simulink model "W_integ_oClientServer_Model"  (R2024b)
settings: Solver=FixedStepDiscrete  StartTime=0.0  StopTime=10.0  FixedStep=0.05  RelTol=1e-3
undefined symbols (not defined in the file or in its folder): call_ServerService_getDataC, call_ServerService_setDataA, call_ServerService_setDataB
settings Model: Tag=EP_AA_WRAPPER_INTEGRATION  DataDictionary=Wrapper_oClientServer_Model.sldd  Creator=nabilekhoury  LastModifiedBy=nabilekhoury
settings OptimizationCC: DefaultParameterBehavior=Inlined  OptimizeBlockIOStorage=off  BufferReuse=off  ReuseModelBlockBuffer=off  GlobalBufferReuse=off  ExpressionFolding=off  EnableMemcpy=off  PassReuseOutputArgsAs=Individual arguments  LocalBlockOutputs=off  ZeroExternalMemoryAtStartup=off  ZeroInternalMemoryAtStartup=off  OptimizeDataStoreBuffers=off  BusAssignmentInplaceUpdate=off  OptimizationLevel=level0  OptimizationCustomize=off  EfficientTunableParamExpr=on
settings DebuggingCC: ParameterTunabilityLossMsg=error
settings ModelReferenceCC: ModelReferenceNumInstancesAllowed=Single
settings SFSimCC: MATLABDynamicMemAlloc=off  SimTargetLang=C++
settings RTWCC: Description=Embedded Coder  SystemTargetFile=ert.tlc  GenCodeOnly=on  TemplateMakefile=ert_default_tmf  CustomSourceCode="#include \"oClientServer_Model_adapter.h\""  CustomInitializer=sut_initialize();  TargetLang=C++
settings CodeAppCC: ForceParamTrailComments=on  IgnoreCustomStorageClasses=off  MaxIdLength=256  OperatorAnnotations=on  SimulinkDataObjDesc=on  SFDataObjDesc=on  CustomSymbolStrGlobalVar=w_$R$N$M  CustomSymbolStrType=w_$N$R$M_T  InsertBlockDesc=on
settings ERTTargetCC: TargetLangStandard=C++17 (ISO)  GenerateSampleERTMain=on  SupportAbsoluteTime=off  SupportNonFinite=off  SupportComplex=off  RootIOFormat=Structure reference  ERTCustomFileTemplate=example_file_process.tlc

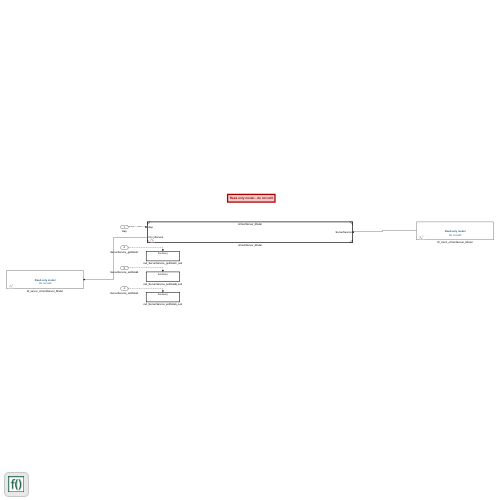
[thumbnail: Simulink's stored preview of the top-level diagram]
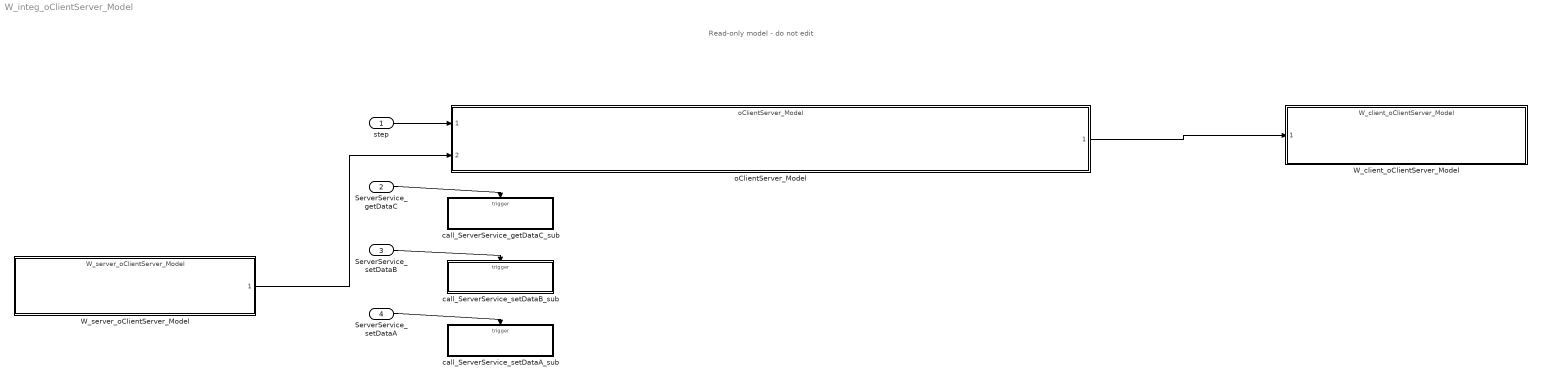
== system W_integ_oClientServer_Model ==
  note: Read-only model - do not edit
  step : Inport  PortDimensions=1  OutputFunctionCall=on
  ServerService_getDataC : Inport  Port=2  OutputFunctionCall=on
  ServerService_setDataB : Inport  Port=3  OutputFunctionCall=on
  ServerService_setDataA : Inport  Port=4  OutputFunctionCall=on
  W_client_oClientServer_Model : ModelReference  ModelNameDialog=W_client_oClientServer_Model  SimulationMode=Normal  ScheduleRates=on  ModelReferenceVersion=1.1
      settings: OpenFcn=open_system(gcb, 'mask');
      mask DialogControl DescGroupVar Prompt: BTC Embedded Systems mocking block
      mask DialogControl DescTextVar Prompt: This is a BTC Embedded Systems mocking block. Do not edit its contents.
      mask Display: disp('\color[rgb]{0.11,0.34,0.51}\bf Read-only model', 'texmode', 'on');disp('\color[rgb]{0.11,0.34,0.51}\newline\newline\rm\it Do not edit', 'texmode', 'on');
  W_server_oClientServer_Model : ModelReference  ModelNameDialog=W_server_oClientServer_Model  SimulationMode=Normal  ScheduleRates=on  ModelReferenceVersion=1.1
      settings: OpenFcn=open_system(gcb, 'mask');
      mask DialogControl DescGroupVar Prompt: BTC Embedded Systems mocking block
      mask DialogControl DescTextVar Prompt: This is a BTC Embedded Systems mocking block. Do not edit its contents.
      mask Display: disp('\color[rgb]{0.11,0.34,0.51}\bf Read-only model', 'texmode', 'on');disp('\color[rgb]{0.11,0.34,0.51}\newline\newline\rm\it Do not edit', 'texmode', 'on');
  call_ServerService_getDataC_sub : Subsystem  TreatAsAtomicUnit=on
  call_ServerService_setDataA_sub : Subsystem  TreatAsAtomicUnit=on
  call_ServerService_setDataB_sub : Subsystem  TreatAsAtomicUnit=on
  oClientServer_Model : ModelReference  Tag=BTC AUTOSAR Main Model Reference Block  ModelNameDialog=oClientServer_Model  SimulationMode=Normal  ScheduleRates=on  ModelReferenceVersion=1.17
  wires:
  step/1 -> oClientServer_Model/1
  W_server_oClientServer_Model/1 -> oClientServer_Model/2
  oClientServer_Model/1 -> W_client_oClientServer_Model/1
  ServerService_getDataC/1 -> call_ServerService_getDataC_sub/Trigger
  ServerService_setDataB/1 -> call_ServerService_setDataB_sub/Trigger
  ServerService_setDataA/1 -> call_ServerService_setDataA_sub/Trigger

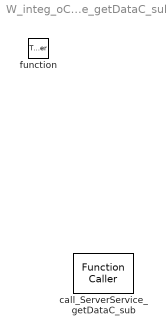
== system W_integ_oClientServer_Model/call_ServerService_getDataC_sub ==
  function : TriggerPort  TriggerType=function-call  VariantControl=(inherit)
  call_ServerService_getDataC_sub : FunctionCaller  FunctionPrototype=call_ServerService_getDataC()  InputArgumentSpecifications=<Enter example>  OutputArgumentSpecifications=<Enter example>

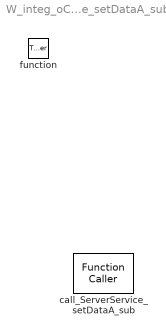
== system W_integ_oClientServer_Model/call_ServerService_setDataA_sub ==
  function : TriggerPort  TriggerType=function-call  VariantControl=(inherit)
  call_ServerService_setDataA_sub : FunctionCaller  FunctionPrototype=call_ServerService_setDataA()  InputArgumentSpecifications=<Enter example>  OutputArgumentSpecifications=<Enter example>

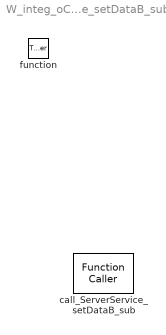
== system W_integ_oClientServer_Model/call_ServerService_setDataB_sub ==
  function : TriggerPort  TriggerType=function-call  VariantControl=(inherit)
  call_ServerService_setDataB_sub : FunctionCaller  FunctionPrototype=call_ServerService_setDataB()  InputArgumentSpecifications=<Enter example>  OutputArgumentSpecifications=<Enter example>
